simulink model "HDLPayloadFull"  (R2024a)
settings: Solver=FixedStepDiscrete  StartTime=0.0  StopTime=stopTime  RelTol=1e-3
values from neighbouring files (symbols this model uses):
  blockSize = logical([0 0])    [testPayloadFull.m]
  dataChars = uint8(zeros(payloadLenInWords, 1))    [testPayloadFull.m]
  fecRate = logical([1 0 0])    [testPayloadFull.m]
  fs = 1    [testPayloadFull.m]
  scramblerInit = logical([1 1 0 0])    [testPayloadFull.m]
libraries: hdlsllib x3, HDL_ieee_8021513 x3, dspsrcs4 x1, whdlutilities x1
settings Model: DataTypeOverride=Off  Creator=cotti  LastModifiedBy=cotti
settings OptimizationCC: BlockReduction=off  ConditionallyExecuteInputs=off  DefaultParameterBehavior=Inlined  InheritOutputTypeSmallerThanSingle=on
settings DebuggingCC: ArtificialAlgebraicLoopMsg=error  SingleTaskRateTransMsg=error
settings HardwareCC: ProdBitPerPointer=32  ProdBitPerSizeT=32  ProdBitPerPtrDiffT=32  ProdLargestAtomicFloat=None  ProdIntDivRoundTo=Undefined  ProdEndianess=Unspecified  ProdWordSize=32  ProdHWDeviceType=ASIC/FPGA->ASIC/FPGA  TargetBitPerLong=64  TargetBitPerPointer=64  TargetBitPerSizeT=64  TargetBitPerPtrDiffT=64  TargetLongLongMode=on  TargetIntDivRoundTo=Zero  TargetEndianess=LittleEndian  TargetWordSize=64  TargetHWDeviceType=Custom Processor->MATLAB Host Computer  ProdEqTarget=off

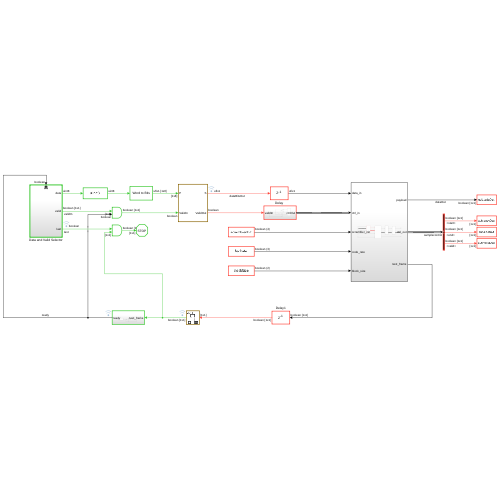
[thumbnail: Simulink's stored preview of the top-level diagram]
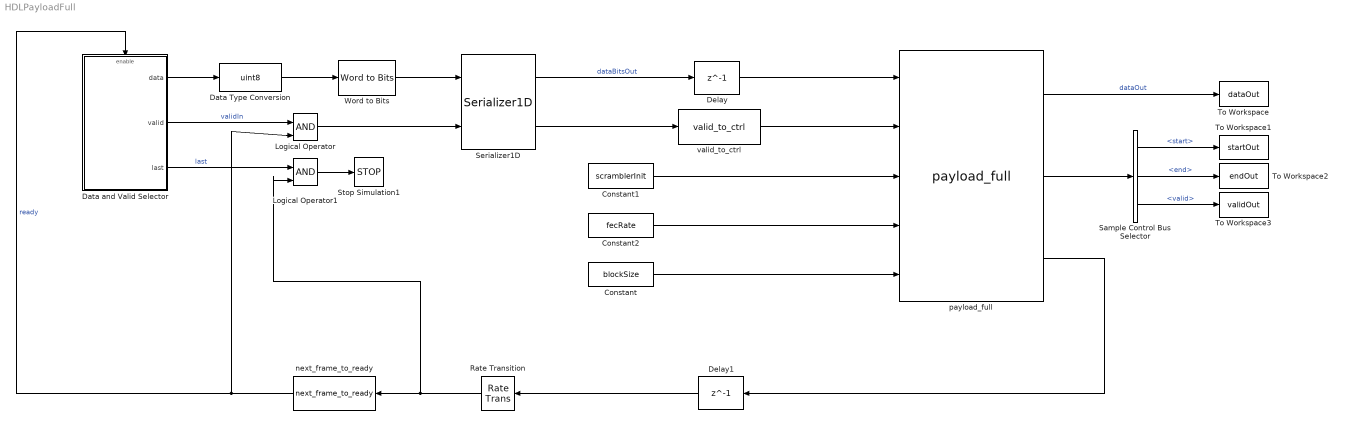
== system HDLPayloadFull ==
  Constant : Constant  Value=blockSize  OutDataTypeStr=boolean  SampleTime=-1
  Constant1 : Constant  Value=scramblerInit  OutDataTypeStr=boolean  SampleTime=-1
  Constant2 : Constant  Value=fecRate  OutDataTypeStr=boolean  SampleTime=-1
  Data Type Conversion : DataTypeConversion  OutDataTypeStr=uint8  SaturateOnIntegerOverflow=off  RndMeth=Floor
  Data and Valid Selector : Subsystem  TreatAsAtomicUnit=on
  Delay : Delay  DelayLength=1  InitialCondition=0  UseCircularBuffer=on
  Delay1 : Delay  DelayLength=1  InitialCondition=0  UseCircularBuffer=on
  Logical Operator : Logic  IconShape=distinctive  AllPortsSameDT=off  OutDataTypeStr=boolean
  Logical Operator1 : Logic  IconShape=distinctive  AllPortsSameDT=off  OutDataTypeStr=boolean
  Rate Transition : RateTransition  OutPortSampleTime=1/fs
  Sample Control Bus Selector : whdlutilities/Sample Control Bus Selector  OutputSignals=start,end,valid
  Serializer1D : hdlsllib/HDL Operations/Serializer1D  Ratio=8  IdleCycles=0  validIn=on  startOut=off  validOut=on  inputDataDimensions=-1  inputSampleTime=-1  inputSignalType=auto
  Stop Simulation1 : Stop
  To Workspace : ToWorkspace  VariableName=dataOut  SampleTime=1/(8*fs)
      settings: Save2DSignal=2-D array (concatenate along first dimension)
  To Workspace1 : ToWorkspace  VariableName=startOut  SampleTime=1/(8*fs)
      settings: Save2DSignal=2-D array (concatenate along first dimension)
  To Workspace2 : ToWorkspace  VariableName=endOut  SampleTime=1/(8*fs)
      settings: Save2DSignal=2-D array (concatenate along first dimension)
  To Workspace3 : ToWorkspace  VariableName=validOut  SampleTime=1/(8*fs)
      settings: Save2DSignal=2-D array (concatenate along first dimension)
  Word to Bits : hdlsllib/Logic and Bit Operations/Word to Bits  maxWordLength=8
  next_frame_to_ready : HDL_ieee_8021513/next_frame_to_ready  SystemSampleTime=-1  VariantActivationTime=update diagram  AllowFlexibleInterface=on  Latency=0  AutoFrameSizeCalculation=off
      settings: SourceProductName=HDL IEEE 8021513
  payload_full : HDL_ieee_8021513/payload_full  SystemSampleTime=-1  VariantActivationTime=update diagram  AllowFlexibleInterface=on  Latency=0  AutoFrameSizeCalculation=off
      settings: SourceProductName=HDL IEEE 8021513
  valid_to_ctrl : HDL_ieee_8021513/valid_to_ctrl  SystemSampleTime=-1  VariantActivationTime=update diagram  AllowFlexibleInterface=on  Latency=0  AutoFrameSizeCalculation=off
      settings: SourceProductName=HDL IEEE 8021513
  wires:
  Sample Control Bus Selector/2 -> To Workspace2/1  "<end>"
  Sample Control Bus Selector/3 -> To Workspace3/1  "<valid>"
  Sample Control Bus Selector/1 -> To Workspace1/1  "<start>"
  payload_full/2 -> Sample Control Bus Selector/1
  payload_full/1 -> To Workspace/1  "dataOut"
  Constant/1 -> payload_full/5
  Constant1/1 -> payload_full/3
  Constant2/1 -> payload_full/4
  Data and Valid Selector/1(data) -> Data Type Conversion/1
  next_frame_to_ready/1 -> Logical Operator/2, Data and Valid Selector/Enable  "ready"
  valid_to_ctrl/1 -> payload_full/2
  Delay/1 -> payload_full/1
  Serializer1D/1 -> Delay/1  "dataBitsOut"
  Serializer1D/2 -> valid_to_ctrl/1
  Data Type Conversion/1 -> Word to Bits/1
  Word to Bits/1 -> Serializer1D/1
  payload_full/3 -> Delay1/1
  Delay1/1 -> Rate Transition/1
  Rate Transition/1 -> Logical Operator1/2, next_frame_to_ready/1
  Data and Valid Selector/2(valid) -> Logical Operator/1  "validIn"
  Logical Operator/1 -> Serializer1D/2
  Data and Valid Selector/3(last) -> Logical Operator1/1  "last"
  Logical Operator1/1 -> Stop Simulation1/1

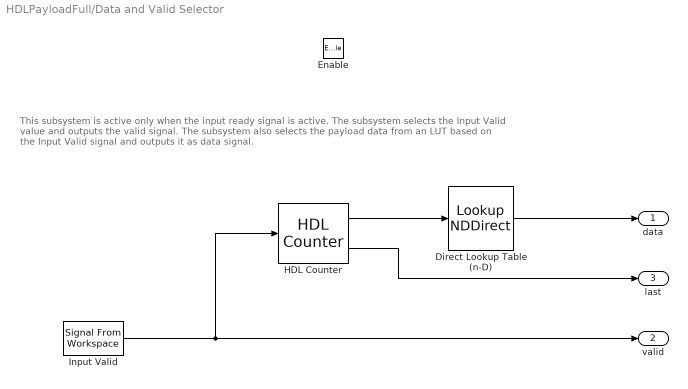
== system HDLPayloadFull/Data and Valid Selector ==
  note: This subsystem is active only when the input ready signal is active. The subsystem selects the Input Valid value and outputs the valid signal.
      | The subsystem also selects the payload data from an LUT based on the Input Valid signal and outputs it as data signal.
  Enable : EnablePort
  Direct Lookup Table (n-D) : LookupNDDirect  NumberOfTableDimensions=1  Table=dataChars  DiagnosticForOutOfRangeInput=Error  TableDataTypeStr=uint8
  HDL Counter : hdlsllib/Sources/HDL Counter  CountType=Count limited  CountInit=0  CountStep=1  CountMax=length(dataChars) -1  CountFromType=Initial value  CountFrom=0  CountResetPort=off  CountLoadPort=off  CountEnbPort=on  CountDirPort=off  CountHitOutputPort=on  CountDataType=Unsigned  CountWordLen=nextpow2(length(dataChars))  CountFracLen=0  CountSampTime=1
  Input Valid : dspsrcs4/Signal From Workspace  X=validIn  Ts=1/fs  nsamps=1  OutputAfterFinalValue=Setting to zero  ignoreOrWarnInputAndFrameLengths=off  OutputFrames=off
  data : Outport  InitialOutput=0  VectorParamsAs1DForOutWhenUnconnected=off
  valid : Outport  Port=2  InitialOutput=0  VectorParamsAs1DForOutWhenUnconnected=off
  last : Outport  Port=3  VectorParamsAs1DForOutWhenUnconnected=off
  wires:
  HDL Counter/1 -> Direct Lookup Table (n-D)/1
  Input Valid/1 -> HDL Counter/1, valid/1
  Direct Lookup Table (n-D)/1 -> data/1
  HDL Counter/2 -> last/1
